simulink model "FaultModel_2022b"  (R2022b)
settings: Solver=ode4  StartTime=0.0  StopTime=inf  FixedStep=0.001  RelTol=1e-3
PreLoadFcn:
  | filepath  = fileparts(get_param(bdroot, 'FileName'));
  | cd(filepath);
InitFcn:
  | Init
values from neighbouring files (symbols this model uses):
  ModelFailEnable = boolean(0)    [Init.m]
  ModelInit_RPM = 0    [Init.m]
  ModelParam_BattHoverMinutes = 18    [Init.m]
  ModelParam_BattHoverThr = 0.609    [Init.m]
  ModelParam_envAltitude = 0    [Init.m]
  ModelParam_GPSEphFinal = 0.3    [Init.m]
  ModelParam_GPSEpvFinal = 0.4    [Init.m]
  ModelParam_GPSFix3DFix = 3    [Init.m]
  ModelParam_GPSSatsVisible = 15    [Init.m]
  ModelParam_motorCr = 1197.53    [Init.m]
  ModelParam_motorJm = 0.0001287    [Init.m]
  ModelParam_motorMinThr = 0.05    [Init.m]
  ModelParam_motorT = 0.02    [Init.m]
  ModelParam_motorWb = 238.2    [Init.m]
  ModelParam_noiseGPSSampTime = 0.02    [Init.m]
  ModelParam_noisePowerIMU = 0    [Init.m]
  ModelParam_noisePowerOffGainAccel = 0.04    [Init.m]
  ModelParam_noisePowerOffGainAccelZ = 0.03    [Init.m]
  ModelParam_noisePowerOffGainGyro = 0.02    [Init.m]
  ModelParam_noisePowerOffGainGyroZ = 0.025    [Init.m]
  ModelParam_noisePowerOffGainMag = 0.02    [Init.m]
  ModelParam_noisePowerOffGainMagZ = 0.035    [Init.m]
  ModelParam_noisePowerOnGainAccel = 0.8    [Init.m]
  ModelParam_noisePowerOnGainAccelZ = 4.5    [Init.m]
  ModelParam_noisePowerOnGainGyro = 2    [Init.m]
  ModelParam_noisePowerOnGainGyroZ = 1    [Init.m]
  ModelParam_noisePowerOnGainMag = 0.025    [Init.m]
  ModelParam_noisePowerOnGainMagZ = 0.05    [Init.m]
  ModelParam_noiseSampleTimeAccel = 0.001    [Init.m]
  ModelParam_noiseSampleTimeGyro = 0.001    [Init.m]
  ModelParam_noiseSampleTimeMag = 0.01    [Init.m]
  ModelParam_rotorCm = 1.779e-07 * adjust_param1    (= 1.4232e-07)    [Init.m]
  ModelParam_rotorCt = 1.105e-05 * adjust_param2    (= 1.6575e-05)    [Init.m]
  ModelParam_timeSampBaro = 0.01    [Init.m]
  ModelParam_uavCCm = [0.0035 0.0039 0.0034]    [Init.m]
  ModelParam_uavCd = [0.7095, 0.6342, 0.9]    [Init.m]
  ModelParam_uavDearo = 0.12    [Init.m]
  ModelParam_uavJ = [ModelParam_uavJxx,0,0;     0,ModelParam_uavJyy,0;     0,0,ModelParam_uavJzz]    [Init.m]
  ModelParam_uavMass = 2.0843    [Init.m]
  ModelParam_uavMotNumbs = int8(4)    [Init.m]
  ModelParam_uavR = 0.225    [Init.m]
  ModelParam_uavType = int8(3)    [Init.m]
undefined symbols (not defined in the file or in its folder): d_i, Earth, F, h_i, Light, MIL, ModelParam_GPSEpvInitial, ModelParam_GPSEpvTimeConstant, ModelParam_noiseLowPassFilterCoeAccel, ModelParam_noiseLowPassFilterCoeGyro, Moderate, Newton, Raphson, WGS84
libraries: simulink x12, aerolibwind2 x3, aerolibtransform2 x3, sharedtransform x3, aerolibasang x3, aerolibatmos2 x2, sharedutil x2, aerolibutil x2, shared6dof x1, aerolibconvert2 x1, aerolibobsolete x1, aerolibnav x1
(part 4 of 4)

== matlab function FaultModel_2022b/Force and Moment Model/Propeller Model old Version ==
  data: uavType input; MotorRads input; R input; uavDearo input; Fb output; Mb output; Cm input; Ct input; Jm input; wb input; Vb input; Cd input; k_ct input
function [Fb,Mb] = fcn(uavType,MotorRads,R,uavDearo,Cm,Ct,Jm,wb,Vb,Cd, k_ct)
% This is control effectiveness model, where Fb is the force produced by motors, Mb is
% the moment produced by motors, and Fd is the resistance produced by the air.
% The gyroscopic torque is not considered here.

% -1: anticlockwise, 1: clockwise 
TypeMotorDirMatrix=[...
    [-1 -1 -1 0 0 0 0 0];... % Tri 3*1 X
    [1 1 1 0 0 0 0 0];...    % Tri 3*1 +
    [-1 -1 1 1 0 0 0 0];... % Quad 4*1 X
    [-1 -1 1 1 0 0 0 0];... % Quad 4*1 +
    [1 -1 1 -1 -1 1 0 0];... % Hex 6*1 X
    [1 -1 1 -1 -1 1 0 0];... % Hex 6*1 +
    [1 -1 1 -1 1 -1 0 0];... % HexCoa 3*2
    [1 1 -1 -1 -1 -1 1 1];... % Oct 8*1 X
    [1 1 -1 -1 -1 -1 1 1];... % Oct 8*1 +
    [1 -1 1 -1 1 -1 1 -1];... % OctCoa 4*2 X
];

TypeMotorAngMatrix=[...
    [pi/3 pi -pi/3 0 0 0 0 0];...
    [pi/3 pi -pi/3 0 0 0 0 0];...
    [pi/4 pi/4+pi pi/4+3*pi/2 pi/4+pi/2 0 0 0 0];...
    [pi/2 3*pi/2 0 pi 0 0 0 0];...
    [pi/2 3/2*pi 3/2*pi+pi/3 pi/2+pi/3 pi/2-pi/3 3/2*pi-pi/3 0 0];...
    [0 pi pi+pi/3 pi/3 -pi/3 pi-pi/3 0 0];...
    [pi/3 pi/3 pi pi -pi/3 -pi/3 0 0];...
    [pi/8 pi+pi/8 pi/8+pi/4 pi-pi/8 -pi/8 3/2*pi-pi/8 3/2*pi+pi/8 pi/2+pi/8];...
    [0 pi pi/4 3/4*pi -pi/4 pi+pi/4 3/2*pi pi/2];...
    [pi/4 -pi/4 pi+pi/4 pi-pi/4 -pi/4 pi/4 pi-pi/4 pi+pi/4];...
];

TypeMotorNonVector=int8([3;3;4;4;6;6;6;8;8;8]);

Mb = [0;0;0];
Fb = [0;0;0];
P=wb(1);Q=wb(2);

if uavType==50
    
    Fb(1)=MotorRads(1)+MotorRads(3);
    Mb(3)=MotorRads(1)*0.1-MotorRads(3)*0.1;
    
    return;
end


if uavType<0||uavType>length(TypeMotorNonVector)
    uavType=int8(1);
end

TypeMotorDirVector=TypeMotorDirMatrix(uavType,:);
TypeMotorAngVector=TypeMotorAngMatrix(uavType,:);

for i=1:TypeMotorNonVector(uavType)
    propAng = TypeMotorAngVector(i);
    propdir = TypeMotorDirVector(i);
    PropT = Ct*MotorRads(i)*MotorRads(i)*k_ct;
    PropM = Cm*MotorRads(i)*MotorRads(i)*k_ct;
    
    %Thrust -> Moment
    Mb=Mb+[-R*sin(propAng)*PropT;R*cos(propAng)*PropT;-PropM*propdir];
    
    %gyroscopic moment
    Mb=Mb+[Q*Jm*MotorRads(i)*propdir;-P*Jm*MotorRads(i)*propdir;0];
    
    Fb=Fb+[0;0;-PropT];
end

 
end

== matlab function FaultModel_2022b/Prop FaultModel/Prop FaultModel/PropFaultModel ==
  settings: updateMethod=DISCRETE
  data: hasFault input; y output; FaultParam input; inPWMs input
function y = fcn(hasFault,FaultParam,inPWMs)
% 本模块需要用到8维FaultParam的输入
%因此故障ID的格式应该是：
%inSILInts=[FaultID FaultID FaultID FaultID ...]
%inSILInts=[param1 param2 param3 param4 param5 param6 param7 param8 ...] -> FaultParam
% param的每一位表示本电机的健康系数（0到1），实际上就是pwm_out = pwm_in * param
% 如果param1=0，则电机1直接坏掉，始终输出0

y=inPWMs; %默认情况下不注入故障，直接将数据输出

if hasFault %如果注入了故障
    for i=1:8
        y(i) = inPWMs(i) * FaultParam(i);
    end
    
end

== matlab function FaultModel_2022b/Battery FaultModel/FaultModelTmp/FaultParamsExtract2 ==
  settings: updateMethod=DISCRETE
  data: FaultID input; inInts input; hasFault_isLowVoltage output; inFloats input; FaultParam output
function [hasFault_isLowVoltage, FaultParam] = fcn(FaultID,inInts,inFloats)
persistent hFault;
persistent fParam;

if isempty(hFault)
    hFault=false;
end
if isempty(fParam)
    fParam=zeros(20,1);
end

hFaultTmp=false;
fParamTmp=zeros(20,1);
j=1;
for i=1:8
    if inInts(i) == FaultID
        hFaultTmp=true;
        fParamTmp(2*j-1)=inFloats(2*i-1);
        fParamTmp(2*j)=inFloats(2*i);
        j=j+1;
    end
end
if hFaultTmp
    hFault=hFaultTmp;
    fParamTmp(17:20) = inFloats(17:20);
    fParam=fParamTmp;
end

hasFault_isLowVoltage=hFault;
FaultParam=fParam;

== matlab function FaultModel_2022b/Battery FaultModel/FaultModelTmp/FaultParamsExtract3 ==
  settings: updateMethod=DISCRETE
  data: FaultID input; inInts input; hasFault_islowCapacity output; inFloats input; FaultParam output
function [hasFault_islowCapacity, FaultParam] = fcn(FaultID,inInts,inFloats)
persistent hFault;
persistent fParam;

if isempty(hFault)
    hFault=false;
end
if isempty(fParam)
    fParam=zeros(20,1);
end

hFaultTmp=false;
fParamTmp=zeros(20,1);
j=1;
for i=1:8
    if inInts(i) == FaultID
        hFaultTmp=true;
        fParamTmp(2*j-1)=inFloats(2*i-1);
        fParamTmp(2*j)=inFloats(2*i);
        j=j+1;
    end
end
if hFaultTmp
    hFault=hFaultTmp;
    fParamTmp(17:20) = inFloats(17:20);
    fParam=fParamTmp;
end

hasFault_islowCapacity=hFault;
FaultParam=fParam;

== matlab function FaultModel_2022b/Fail Model/Prop FaultModel/FaultParamsExtract3 ==
  settings: updateMethod=DISCRETE
  data: FaultID input; inInts input; hasFault_isloadFall output; inFloats input; FaultParam output
function [hasFault_isloadFall, FaultParam] = fcn(FaultID,inInts,inFloats)
persistent hFault;
persistent fParam;

if isempty(hFault)
    hFault=false;
end
if isempty(fParam)
    fParam=zeros(20,1);
end

hFaultTmp=false;
fParamTmp=zeros(20,1);
j=1;
for i=1:8
    if inInts(i) == FaultID
        hFaultTmp=true;
        fParamTmp(2*j-1)=inFloats(2*i-1);
        fParamTmp(2*j)=inFloats(2*i);
        j=j+1;
    end
end
if hFaultTmp
    hFault=hFaultTmp;
    fParamTmp(17:20) = inFloats(17:20);
    fParam=fParamTmp;
end

hasFault_isloadFall=hFault;
FaultParam=fParam;

== matlab function FaultModel_2022b/Fail Model/Prop FaultModel/FaultParamsExtract2 ==
  settings: updateMethod=DISCRETE
  data: FaultID input; inInts input; hasFault_isloadLeak output; inFloats input; FaultParam output
function [hasFault_isloadLeak, FaultParam] = fcn(FaultID,inInts,inFloats)
persistent hFault;
persistent fParam;

if isempty(hFault)
    hFault=false;
end
if isempty(fParam)
    fParam=zeros(20,1);
end

hFaultTmp=false;
fParamTmp=zeros(20,1);
j=1;
for i=1:8
    if inInts(i) == FaultID
        hFaultTmp=true;
        fParamTmp(2*j-1)=inFloats(2*i-1);
        fParamTmp(2*j)=inFloats(2*i);
        j=j+1;
    end
end
if hFaultTmp
    hFault=hFaultTmp;
    fParamTmp(17:20) = inFloats(17:20);
    fParam=fParamTmp;
end

hasFault_isloadLeak=hFault;
FaultParam=fParam;

== matlab function FaultModel_2022b/Environment FaultModel1/Env FaultWindModel/FaultParamsExtract ==
  settings: updateMethod=DISCRETE
  data: FaultID input; inInts input; hasFault_ConstWind output; inFloats input; FaultParam output
function [hasFault_ConstWind, FaultParam] = fcn(FaultID,inInts,inFloats)
persistent hFault;
persistent fParam;

if isempty(hFault)
    hFault=false;
end
if isempty(fParam)
    fParam=zeros(20,1);
end

hFaultTmp=false;
fParamTmp=zeros(20,1);
j=1;
for i=1:8
    if inInts(i) == FaultID
        hFaultTmp=true;
        fParamTmp(2*j-1)=inFloats(2*i-1);
        fParamTmp(2*j)=inFloats(2*i);
        j=j+1;
    end
end
if hFaultTmp
    hFault=hFaultTmp;
    fParamTmp(17:20) = inFloats(17:20);
    fParam=fParamTmp;
end

hasFault_ConstWind=hFault;
FaultParam=fParam;

== matlab function FaultModel_2022b/Environment FaultModel1/Env FaultWindModel/FaultParamsExtract2 ==
  settings: updateMethod=DISCRETE
  data: FaultID input; inInts input; hasFault_TurbWind output; inFloats input; FaultParam output
function [hasFault_TurbWind, FaultParam] = fcn(FaultID,inInts,inFloats)
persistent hFault;
persistent fParam;

if isempty(hFault)
    hFault=false;
end
if isempty(fParam)
    fParam=zeros(20,1);
end

hFaultTmp=false;
fParamTmp=zeros(20,1);
j=1;
for i=1:8
    if inInts(i) == FaultID
        hFaultTmp=true;
        fParamTmp(2*j-1)=inFloats(2*i-1);
        fParamTmp(2*j)=inFloats(2*i);
        j=j+1;
    end
end
if hFaultTmp
    hFault=hFaultTmp;
    fParamTmp(17:20) = inFloats(17:20);
    fParam=fParamTmp;
end

hasFault_TurbWind=hFault;
FaultParam=fParam;

== matlab function FaultModel_2022b/Environment FaultModel1/Env FaultWindModel/FaultParamsExtract3 ==
  settings: updateMethod=DISCRETE
  data: FaultID input; inInts input; hasFault_SheerWind output; inFloats input; FaultParam output
function [hasFault_SheerWind, FaultParam] = fcn(FaultID,inInts,inFloats)
persistent hFault;
persistent fParam;

if isempty(hFault)
    hFault=false;
end
if isempty(fParam)
    fParam=zeros(20,1);
end

hFaultTmp=false;
fParamTmp=zeros(20,1);
j=1;
for i=1:8
    if inInts(i) == FaultID
        hFaultTmp=true;
        fParamTmp(2*j-1)=inFloats(2*i-1);
        fParamTmp(2*j)=inFloats(2*i);
        j=j+1;
    end
end
if hFaultTmp
    hFault=hFaultTmp;
    fParamTmp(17:20) = inFloats(17:20);
    fParam=fParamTmp;
end

hasFault_SheerWind=hFault;
FaultParam=fParam;

== matlab function FaultModel_2022b/OutputPort1/HILSensorMavModel1/Subsystem/baro NoiseFun ==
  data: noise input; isbyroFault input; y output; baroFaultParam input; y_sacle output
function [y, y_sacle] = fcn(noise, isbyroFault,baroFaultParam)
y = 0;
y_scale = [1,1,1];

if isbyroFault
    if baroFaultParam(1) == 3
        y = (0.2+0.8*baroFaultParams(3)) * noise + baroFaultParams(2);
    elseif baroFaultParam(1) == 4
        y_scale = baroFaultParam(2);
    end
end

== matlab function FaultModel_2022b/OutputPort1/HILGPSModel/AccNoiseSwitch1/Acc NoiseFun ==
  data: u input; y output; isAccFault input; AccFaultParams input; y_scale output
function [y, y_scale] = fcn(u,isAccFault,AccFaultParams)

y = 0.3*u;
y_scale = [1,1,1];

if isAccFault
    if AccFaultParams(1) == 3
        y = [0.3+0.7*AccFaultParams(3), 0.3+0.7*AccFaultParams(5),0.3+0.7*AccFaultParams(7)] .*u + [AccFaultParams(2),AccFaultParams(4),AccFaultParams(6)];
        % y = (0.2+0.8*AccFaultParams(2))*u;
    elseif AccFaultParams(1) == 4
        y_scale = [AccFaultParams(2), AccFaultParams(3), AccFaultParams(4)];
    end
end

== matlab function FaultModel_2022b/Motor FaultModel/FaultModelTmp/MATLAB Function ==
  data: isnoMotorProFault input; y output; isMotorProFault input; inPWMs input; NoProPWMOut input; ProPWMOut input
function y = fcn(isnoMotorProFault,isMotorProFault,inPWMs,NoProPWMOut,ProPWMOut)

y = inPWMs;
if isnoMotorProFault
   y =  NoProPWMOut;
elseif isMotorProFault
   y = ProPWMOut;
end

== matlab function FaultModel_2022b/Motor FaultModel/FaultModelTmp/motor_fauilure_protection ==
  data: hasFault input; FaultParams input; inPWMs input; y output; count input
function y = fcn(hasFault,FaultParams,inPWMs,count)
y=inPWMs;
if hasFault %如果注入了故障(自旋下降处理)
    if count == 1
        y(1) = inPWMs(1) * FaultParams(1);
        y(2) = inPWMs(2) * FaultParams(2);
        if FaultParams(1)==0
            y(3)=0.835;
            y(4)=0.835;
            y(2)=0;
        end
        if FaultParams(2)==0
            y(1)=0;
            y(3)=0.835;
            y(4)=0.835;
        end
    elseif count == 2
        for i=1:4
            y(i) = inPWMs(i) * FaultParams(i);
        end
        if FaultParams(1)==0
            y(3)=0.835;
            y(4)=0.835;
            y(2)=0;
        end
        if FaultParams(2)==0
            y(1)=0;
            y(3)=0.835;
            y(4)=0.835;
        end
        if FaultParams(3)==0
            y(4)=0;
            y(1)=0.835;
            y(2)=0.835;
        end
        if FaultParams(4)==0
            y(3)=0;
            y(1)=0.835;
            y(2)=0.835;
        end
    end
end


%     if inSILFloats(1)==0
%         y(2)=y(2)-0.25;
%     end
%     if inSILFloats(2)==0
%         y(1)=y(1)-0.25;
%     end
%     if inSILFloats(3)==0
%         y(4)=y(4)-0.25;
%     end
%     if inSILFloats(4)==0
%         y(3)=y(3)-0.25;
%     end
% 
% if inSILInts(1)==3 %坠机就令PWM为0
%     y(1)=0;
%     y(2)=0;
%     y(3)=0;
%     y(4)=0;
% end

== matlab function FaultModel_2022b/Force and Moment Model/Ground Model ==
  settings: updateMethod=DISCRETE
  data: mg input; wb input; Xe input; F1 output; Ve input; M1 output; Quet input; terrainZ input; landed output; takeoff output
function [F1,M1,landed,takeoff] = fcn(mg,wb,Xe,Ve,Quet,terrainZ)
% This is a ground model that can provides reaction force and reaction torque

% persistent z0;
% if isempty(z0)
%      z0=0;
% end

persistent takeoffFlag;
if isempty(takeoffFlag)
     takeoffFlag=int8(0);
end

persistent landFlag;
if isempty(landFlag)
     landFlag=int8(1);
end

z=Xe(3)-terrainZ;

if (z<-0.3)&&(Ve(3)<-0.1)&&(takeoffFlag<0.5)
    takeoffFlag=int8(1);
    landFlag=int8(0);
end

if (z>-0.05)&&(Ve(3)>0.1)&&(landFlag<0.5)
    landFlag=int8(1);
    takeoffFlag=int8(0);
end

takeoff = takeoffFlag;
landed = landFlag;


F1=[0;0;0];
M1=[0;0;0];

if z>=0
%     if z>=0.3
%         if Ve(3)>=5
%             F1(3)=-mg(3)-1000*Ve(3);
%         else
%             F1(3)=-mg(3)-500*z-100*Ve(3);  
%         end
%     elseif z>=0.1
%         if Ve(3)>=2
%             F1(3)=-mg(3)-100*Ve(3);
%         else
%             F1(3)=-mg(3)-50*z-100*Ve(3);  
%         end
%     else
%          if Ve(3)>=1
%             F1(3)=-mg(3)-50*Ve(3);
%         else
%             F1(3)=-mg(3)-5*z-50*Ve(3);  
%         end       
%     end
    if z<0.05
        F1(3)=-mg(3)-10*Ve(3); 
    elseif z<0.1
        F1(3)=-mg(3)-0.5*z-20*Ve(3); 
    else
        F1(3)=-mg(3)-1*z-50*Ve(3); 
    end

    F1(1)=-50*Ve(1);
    F1(2)=-50*Ve(2);
    
%     if ~(isnan(Quet(2))||isnan(Quet(3))||isnan(Quet(4)))
%         M1=-200*[Quet(2);Quet(3);Quet(4)]-10*wb;
%     end
    
    M1=-20*[Quet(2);Quet(3);Quet(4)]-5*wb;
    M1 = M1 * abs(mg(3))*0.0333;
end

== matlab function FaultModel_2022b/Battery FaultModel/FaultModelTmp/FaultParamsExtract ==
  settings: updateMethod=DISCRETE
  data: FaultID input; inInts input; hasFault_isUseCustomHovTime output; inFloats input; FaultParam output
function [hasFault_isUseCustomHovTime, FaultParam] = fcn(FaultID,inInts,inFloats)
persistent hFault;
persistent fParam;

if isempty(hFault)
    hFault=false;
end
if isempty(fParam)
    fParam=zeros(20,1);
end

hFaultTmp=false;
fParamTmp=zeros(20,1);
j=1;
for i=1:8
    if inInts(i) == FaultID
        hFaultTmp=true;
        fParamTmp(2*j-1)=inFloats(2*i-1);
        fParamTmp(2*j)=inFloats(2*i);
        j=j+1;
    end
end
if hFaultTmp
    hFault=hFaultTmp;
    fParamTmp(17:20) = inFloats(17:20);
    fParam=fParamTmp;
end

hasFault_isUseCustomHovTime=hFault;
FaultParam=fParam;

== matlab function FaultModel_2022b/Force and Moment Model/Prop FaultModel/Prop FaultModel/FaultParamsExtract ==
  settings: updateMethod=DISCRETE
  data: FaultID input; inInts input; hasFault output; inFloats input; FaultParam output
function [hasFault, FaultParam] = fcn(FaultID,inInts,inFloats)
persistent hFault;
persistent fParam;

if isempty(hFault)
    hFault=false;
end
if isempty(fParam)
    fParam=zeros(20,1);
end

hFaultTmp=false;
fParamTmp=zeros(20,1);
j=1;
for i=1:8
    if inInts(i) == FaultID
        hFaultTmp=true;
        fParamTmp(2*j-1)=inFloats(2*i-1);
        fParamTmp(2*j)=inFloats(2*i);
        j=j+1;
    end
end
if hFaultTmp
    hFault=hFaultTmp;
    fParamTmp(17:20) = inFloats(17:20);
    fParam=fParamTmp;
end

hasFault=hFault;
FaultParam=fParam;
